simulink model "MOD2"  (R2016a)
settings: Solver=FixedStepAuto  StartTime=0.0  StopTime=0.1  RelTol=1e-3
undefined symbols (not defined in the file): a, b
libraries: dspmlti4 x4, dsparch4 x1
settings Model: Creator=bhannigan  LastModifiedBy=bhannigan

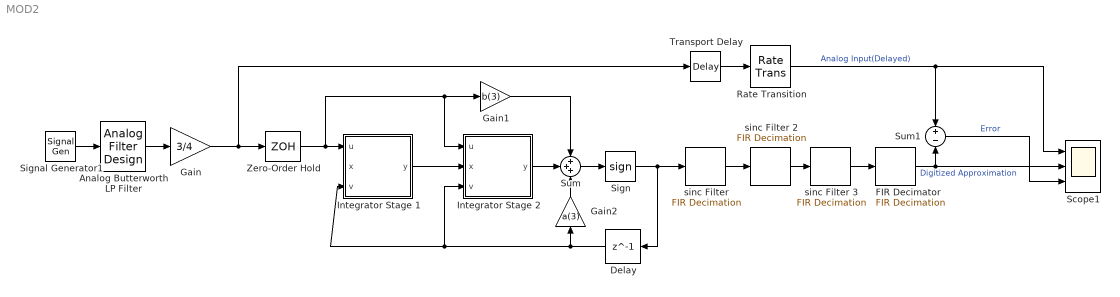
== system MOD2 ==
  Analog Butterworth LP Filter : dsparch4/Analog Filter Design  method=Butterworth  filttype=Lowpass  N=5  Wlo=2*pi*400  Whi=80  Rp=2  Rs=40
  Delay : Delay  DelayLength=1  InitialCondition=0
  FIR Decimator : dspmlti4/FIR Decimation  FilterSource=Dialog parameters  h=fir1(63, 0.25)  D=4  filtStruct=Direct form  FilterObject=Hm_firdecim  framing=Allow multirate processing  inputOffset=0  outputBufInitCond=0  roundingMode=Floor  overflowMode=off  firstCoeffDataTypeStr=Inherit: Same word length as input  firstCoeffMin=[]  firstCoeffMax=[]  firstCoeffLastDataTypeStr=Inherit: Same word length as input  accumDataTypeStr=Inherit: Same as product output  accumLastDataTypeStr=Inherit: Same as product output  outputMin=[]  outputMax=[]
  Gain : Gain  Gain=3/4  SaturateOnIntegerOverflow=on  OutDataTypeStr=Inherit: Same as input  ParamDataTypeStr=Inherit: Same as input
  Gain1 : Gain  Gain=b(3)
  Gain2 : Gain  Gain=a(3)
  Integrator Stage 1 : Subsystem  mask{a=a(1), b=b(1)}
      mask prompts: a "Feedback gain:"; b "Feedforward gain:"
  Integrator Stage 2 : Subsystem  mask{a=a(1), b=b(1)}
      mask prompts: a "Feedback gain:"; b "Feedforward gain:"
  Rate Transition : RateTransition
  Scope1 : Scope  NumInputPorts=3
  Sign : Signum
  Signal Generator1 : SignalGenerator  WaveForm=square  Frequency=80
  Sum : Sum  Inputs=+++
  Sum1 : Sum  Inputs=+-  SaturateOnIntegerOverflow=on  InputSameDT=on  OutDataTypeStr=Inherit: Same as first input
  Transport Delay : TransportDelay  DelayTime=736/512000
  Zero-Order Hold : ZeroOrderHold  SampleTime=1/512000
  sinc Filter : dspmlti4/FIR Decimation  FilterSource=Dialog parameters  h=1/64*ones(1, 64)  D=2  filtStruct=Direct form  FilterObject=Hm_firdecim  framing=Allow multirate processing  inputOffset=0  outputBufInitCond=0  roundingMode=Floor  overflowMode=off  firstCoeffDataTypeStr=Inherit: Same word length as input  firstCoeffMin=[]  firstCoeffMax=[]  firstCoeffLastDataTypeStr=Inherit: Same word length as input  accumDataTypeStr=Inherit: Same as product output  accumLastDataTypeStr=Inherit: Same as product output  outputMin=[]  outputMax=[]
  sinc Filter 2 : dspmlti4/FIR Decimation  FilterSource=Dialog parameters  h=1/64*ones(1, 64)  D=2  filtStruct=Direct form  FilterObject=Hm_firdecim  framing=Allow multirate processing  inputOffset=0  outputBufInitCond=0  roundingMode=Floor  overflowMode=off  firstCoeffDataTypeStr=Inherit: Same word length as input  firstCoeffMin=[]  firstCoeffMax=[]  firstCoeffLastDataTypeStr=Inherit: Same word length as input  accumDataTypeStr=Inherit: Same as product output  accumLastDataTypeStr=Inherit: Same as product output  outputMin=[]  outputMax=[]
  sinc Filter 3 : dspmlti4/FIR Decimation  FilterSource=Dialog parameters  h=1/64*ones(1, 64)  D=4  filtStruct=Direct form  FilterObject=Hm_firdecim  framing=Allow multirate processing  inputOffset=0  outputBufInitCond=0  roundingMode=Floor  overflowMode=off  firstCoeffDataTypeStr=Inherit: Same word length as input  firstCoeffMin=[]  firstCoeffMax=[]  firstCoeffLastDataTypeStr=Inherit: Same word length as input  accumDataTypeStr=Inherit: Same as product output  accumLastDataTypeStr=Inherit: Same as product output  outputMin=[]  outputMax=[]
  wires:
  Analog Butterworth LP Filter/1 -> Gain/1
  Signal Generator1/1 -> Analog Butterworth LP Filter/1
  Integrator Stage 1/1(y) -> Integrator Stage 2/2(x)
  Gain/1 -> Transport Delay/1, Zero-Order Hold/1
  Sum/1 -> Sign/1
  Gain1/1 -> Sum/1
  Delay/1 -> Gain2/1, Integrator Stage 2/3(v), Integrator Stage 1/3(v)
  Sum1/1 -> Scope1/3  "Error"
  Transport Delay/1 -> Rate Transition/1
  Sign/1 -> sinc Filter/1, Delay/1
  Zero-Order Hold/1 -> Integrator Stage 2/1(u), Gain1/1, Integrator Stage 1/1(u)
  Rate Transition/1 -> Scope1/1, Sum1/1  "Analog Input(Delayed)"
  Gain2/1 -> Sum/3
  sinc Filter 2/1 -> sinc Filter 3/1
  sinc Filter/1 -> sinc Filter 2/1
  sinc Filter 3/1 -> FIR Decimator/1
  FIR Decimator/1 -> Scope1/2, Sum1/2  "Digitized Approximation"
  Integrator Stage 2/1(y) -> Sum/2

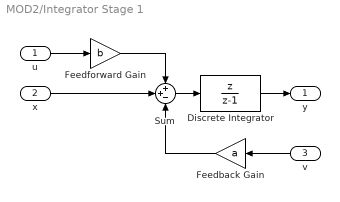
== system MOD2/Integrator Stage 1 ==
  u : Inport
  x : Inport  Port=2
  v : Inport  Port=3
  Discrete Integrator : DiscreteTransferFcn  Numerator=[1 0]  Denominator=[1 -1]
  Feedback Gain : Gain  Gain=a
  Feedforward Gain : Gain  Gain=b
  Sum : Sum  Inputs=++-
  y : Outport
  wires:
  x/1 -> Sum/2
  Sum/1 -> Discrete Integrator/1
  Feedback Gain/1 -> Sum/3
  Feedforward Gain/1 -> Sum/1
  u/1 -> Feedforward Gain/1
  v/1 -> Feedback Gain/1
  Discrete Integrator/1 -> y/1

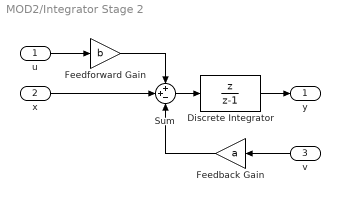
== system MOD2/Integrator Stage 2 ==
  u : Inport
  x : Inport  Port=2
  v : Inport  Port=3
  Discrete Integrator : DiscreteTransferFcn  Numerator=[1 0]  Denominator=[1 -1]
  Feedback Gain : Gain  Gain=a
  Feedforward Gain : Gain  Gain=b
  Sum : Sum  Inputs=++-
  y : Outport
  wires:
  x/1 -> Sum/2
  Sum/1 -> Discrete Integrator/1
  Feedback Gain/1 -> Sum/3
  Feedforward Gain/1 -> Sum/1
  u/1 -> Feedforward Gain/1
  v/1 -> Feedback Gain/1
  Discrete Integrator/1 -> y/1
